simulink model "mapp_4_fir_4_str"  (R2018b)
settings: Solver=ode45  StartTime=0.0  StopTime=200  RelTol=1e-3  EnableMultiTasking=on
undefined symbols (not defined in the file or in its folder): CMD_ci_Re_0, CMD_ci_Re_21, CMD_ci_str_0, CMD_ci_str_1, CMD_ci_str_10, CMD_ci_str_11, CMD_ci_str_12, CMD_ci_str_13, CMD_ci_str_14, CMD_ci_str_15, CMD_ci_str_16, CMD_ci_str_17, CMD_ci_str_18, CMD_ci_str_19, CMD_ci_str_2, CMD_ci_str_20, CMD_ci_str_21, CMD_ci_str_3, CMD_ci_str_4, CMD_ci_str_5, CMD_ci_str_6, CMD_ci_str_7, CMD_ci_str_8, CMD_ci_str_9, CMD_decr_0, CMD_deka_down, CMD_deka_up, CMD_fb, CMD_FB_mult, CMD_Firprg_0, CMD_Firprg_1, CMD_gain, CMD_ind_mult, CMD_ind_mult_1, CMD_ind_mult_2, CMD_ind_mult_3, CMD_ind_mult_4, CMD_ind_stuk, CMD_ind_vol, CMD_ind_vol_1, CMD_ind_vol_2, CMD_ind_vol_3, CMD_ind_vol_4, CMD_init_dac, CMD_init_sw, CMD_molot_string, CMD_nl, CMD_nl_sl, CMD_omega_0, CMD_out_vol, CMD_param_0, CMD_param_5, CMD_pedal, CMD_reset, CMD_rst, CMD_shape_0, CMD_step_down, CMD_step_up, CMD_str_svertk, ind_mult_0 ... (+10)
libraries: xbsIndex_r4 x3300
(part 16 of 16)

== system mapp_4_fir_4_str/mashinka_0/Force_str0/PARAMETERS/Subsystem1/Subsystem1 ==
  In1 : Inport
  Convert : xbsIndex_r4/Convert  gui_display_data_type=Boolean  arith_type=Boolean  n_bits=16  bin_pt=14  float_type=Single  exp_bits=8  fraction_bits=24  quantization=Truncate  overflow=Wrap  en=off  latency=0  pipeline=off  dbl_ovrd=off  block_type=convert
  Delay8 : xbsIndex_r4/Delay  rst=off  infoeditControl=Selection of Reset will increase slice count due to use of real FFs and instead of SRLs  en=off  latency=1  reg_retiming=off  dbl_ovrd=off  block_type=delay
  Delay9 : xbsIndex_r4/Delay  rst=off  infoeditControl=Selection of Reset will increase slice count due to use of real FFs and instead of SRLs  en=off  latency=1  reg_retiming=off  dbl_ovrd=off  block_type=delay
  Logical : xbsIndex_r4/Logical  logical_function=XOR  inputs=2  en=off  latency=0  precision=Full  arith_type=Unsigned  n_bits=16  bin_pt=0  align_bp=on  dbl_ovrd=off  block_type=logical
  Logical1 : xbsIndex_r4/Logical  logical_function=AND  inputs=2  en=off  latency=0  precision=Full  arith_type=Unsigned  n_bits=16  bin_pt=0  align_bp=on  dbl_ovrd=off  block_type=logical
  Logical2 : xbsIndex_r4/Logical  logical_function=AND  inputs=2  en=off  latency=0  precision=Full  arith_type=Unsigned  n_bits=16  bin_pt=0  align_bp=on  dbl_ovrd=off  block_type=logical
  Scope1 : Scope  NumInputPorts=8
  rise : Outport
  fall : Outport  Port=2
  wires:
  Convert/1 -> Logical1/1, Scope1/1, Delay9/1, Logical/1
  Delay9/1 -> Logical2/2, Logical/2
  Logical/1 -> Logical2/1, Logical1/2
  Logical1/1 -> Scope1/2, rise/1
  Logical2/1 -> Scope1/3, fall/1
  In1/1 -> Delay8/1
  Delay8/1 -> Convert/1

== system mapp_4_fir_4_str/mashinka_0/Force_str0/PARAMETERS/Subsystem1/en1 ==
  In1 : Inport
  Delay : xbsIndex_r4/Delay  rst=off  infoeditControl=Selection of Reset will increase slice count due to use of real FFs and instead of SRLs  en=off  latency=1  reg_retiming=off  dbl_ovrd=off  block_type=delay
  Logical : xbsIndex_r4/Logical  logical_function=AND  inputs=2  en=off  latency=0  precision=Full  arith_type=Unsigned  n_bits=16  bin_pt=0  align_bp=on  dbl_ovrd=off  block_type=logical
  Logical1 : xbsIndex_r4/Logical  logical_function=XOR  inputs=2  en=off  latency=0  precision=Full  arith_type=Unsigned  n_bits=16  bin_pt=0  align_bp=on  dbl_ovrd=off  block_type=logical
  Out1 : Outport
  wires:
  In1/1 -> Logical/1, Delay/1, Logical1/2
  Logical/1 -> Out1/1
  Delay/1 -> Logical1/1
  Logical1/1 -> Logical/2
